simulink model "simulation_poleplacement_azioneintegrale_WP2_L"  (R2023b)
settings: Solver=VariableStepAuto  StartTime=0.0  StopTime=20  RelTol=1e-3
values from neighbouring files (symbols this model uses):
  A = [0 1; 9.81 -0.1]    [WP2.m]
  B = [0; 1]    [WP2.m]
  K = [k1 k2 ki]    [WP2.m]
  rl = 0    [WP2.m]
settings Model: Creator=giova  LastModifiedBy=miche

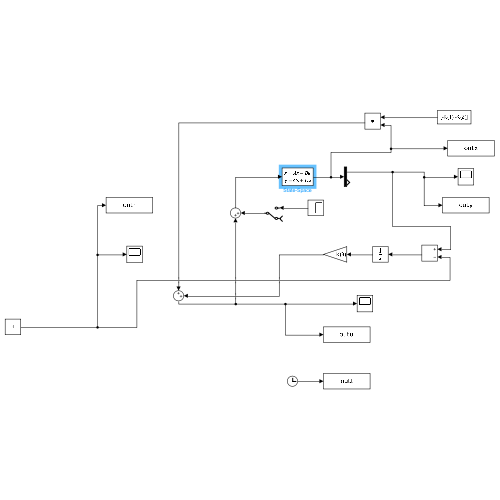
[thumbnail: Simulink's stored preview of the top-level diagram]
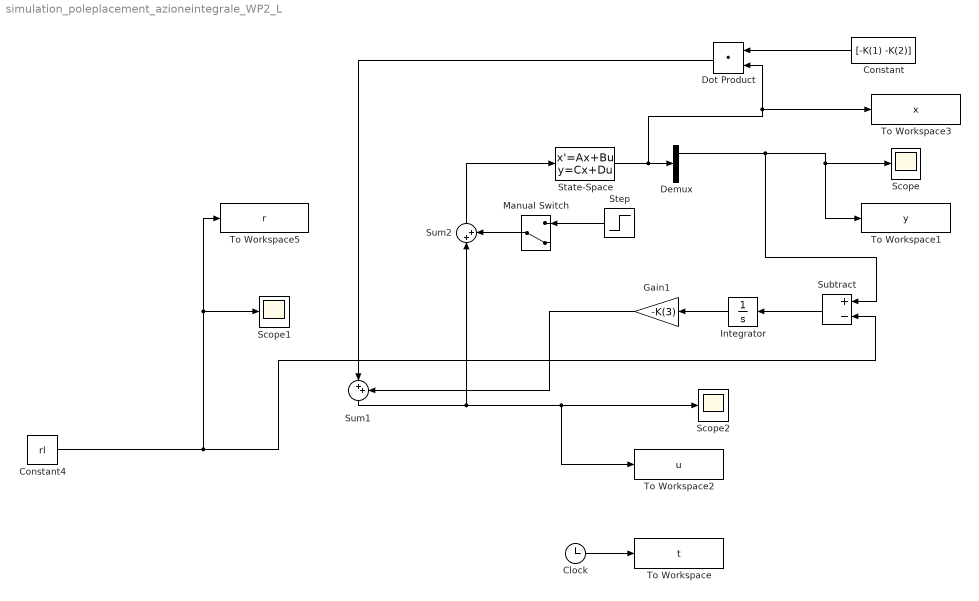
== system simulation_poleplacement_azioneintegrale_WP2_L ==
  Clock : Clock
  Constant : Constant  Value=[-K(1) -K(2)]
  Constant4 : Constant  Value=rl
  Demux : Demux  Outputs=2
  Dot Product : DotProduct  OutDataTypeStr=Inherit: Inherit via internal rule
  Gain1 : Gain  Gain=-K(3)
  Integrator : Integrator
  Manual Switch : ManualSwitch  CurrentSetting=0
  Scope : Scope
  Scope1 : Scope
  Scope2 : Scope
  State-Space : StateSpace  A=A  B=B  C=eye(2)  D=[0;0]  InitialCondition=[pi, 0]
  Step : Step  Time=5  After=10000  SampleTime=0
  Subtract : Sum  Inputs=+-
  Sum1 : Sum  Inputs=|++
  Sum2 : Sum  Inputs=|++
  To Workspace : ToWorkspace  VariableName=t  SampleTime=-1
  To Workspace1 : ToWorkspace  VariableName=y  SampleTime=-1
  To Workspace2 : ToWorkspace  VariableName=u  SampleTime=-1
  To Workspace3 : ToWorkspace  VariableName=x  SampleTime=-1
  To Workspace5 : ToWorkspace  VariableName=r  SampleTime=-1
  wires:
  Sum1/1 -> Sum2/1, Scope2/1, To Workspace2/1
  Clock/1 -> To Workspace/1
  Constant/1 -> Dot Product/1
  State-Space/1 -> To Workspace3/1, Dot Product/2, Demux/1
  Demux/1 -> Subtract/1, To Workspace1/1, Scope/1
  Dot Product/1 -> Sum1/1
  Subtract/1 -> Integrator/1
  Integrator/1 -> Gain1/1
  Constant4/1 -> Scope1/1, To Workspace5/1, Subtract/2
  Gain1/1 -> Sum1/2
  Sum2/1 -> State-Space/1
  Manual Switch/1 -> Sum2/2
  Step/1 -> Manual Switch/1
